simulink model "DFT_Stream_Ex1"  (R2022a)
settings: Solver=VariableStepAuto  StartTime=0.0  StopTime=0.6  RelTol=1e-3
undefined symbols (not defined in the file): None, S, vsva2197, xcvc1902
libraries: dspsrcs4 x1, aieDSP x1, vmcUtilities x1
settings Model: Creator=sdegala  LastModifiedBy=sdegala

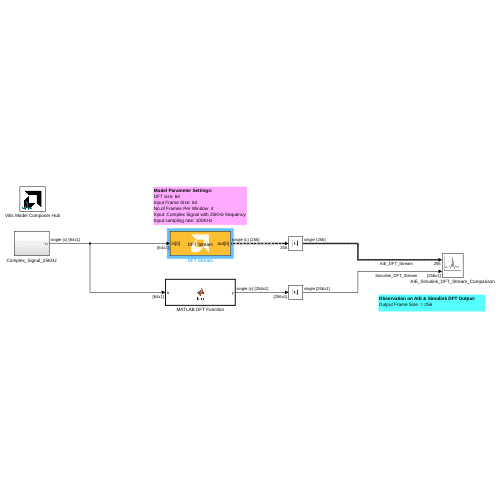
[thumbnail: Simulink's stored preview of the top-level diagram]
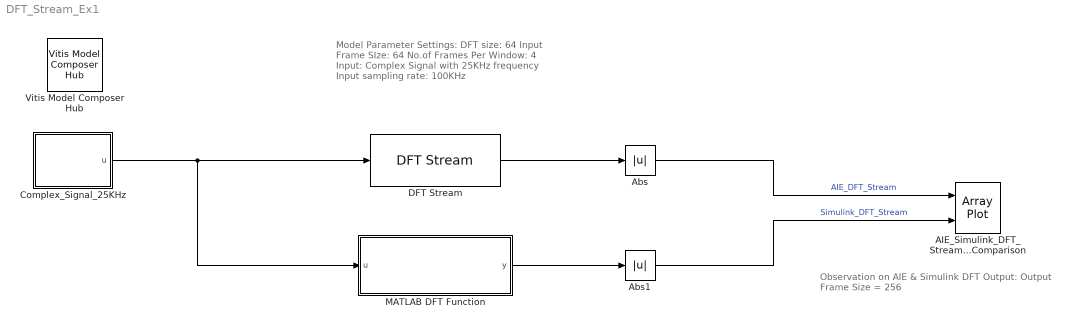
== system DFT_Stream_Ex1 ==
  note: Model Parameter Settings:
      | DFT size: 64
      | Input Frame SIze: 64
      | No.of Frames Per Window: 4
      | Input: Complex Signal with 25KHz frequency
      | Input sampling rate: 100KHz
  note: Observation on AIE & Simulink DFT Output:
      | Output Frame Size = 256
  AIE_Simulink_DFT_Stream_Comparison : ArrayPlot  NumInputPorts=2  WindowPosition=[5.000000,41.000000,1272.000000,651.000000,]  ScopeFrameLocation=window  YLimits=[-80,720]  ShowLegend=on
  Abs : Abs  SaturateOnIntegerOverflow=off
  Abs1 : Abs  SaturateOnIntegerOverflow=off
  Complex_Signal_25KHz : Subsystem
  DFT Stream : aieDSP/DFT Stream  data_type=cfloat  twiddle_type=cfloat  point_size=64  num_frames=4  shift_val=0  rnd_mode=Round symmetrical to infinity  sat_mode=0-None  casc_length=1  blockJsonConstraints=[]  blockJsonConstraintsInternal=[]  spec=vmc_stream_dft.json  SerializedMaskParamNames=[]  SerializedMaskParamValues=[]  SerializedMaskParamVisibilities=[]  block_type=DFT Stream  SerializedMaskParamDataypes=typename|typename|uint|uint|uint|uint|uint|uint  SerializedMaskParamEnumStrArr=0|0|0|0|0|Floor,Ceiling,Round to positive infinity,Round to negative infinity,Round symmetrical to infinity,Round symmetrical to zero,Round convergent to even,Round convergent to odd|0-None,1-Asymmetric,3-Symmetric|0  SerializedMaskParamEnumValArr=0|0|0|0|0|0,1,2,3,4,5,6,7|0,1,3|0  SerializedMaskParamVectorArr=0|0|0|0|0|0|0|0
  MATLAB DFT Function : MATLAB Function  TreatAsAtomicUnit=on
  Vitis Model Composer Hub : vmcUtilities/Vitis Model Composer Hub  Tag=genX  CodeGeneration=off  TargetDirectory=./code  ExportType=AI Engines  IpVendor=xilinx.com  IpLibrary=hls  IpVersion=1.0  IpHWLanguage=Verilog  AieCompilerOptions={}  AieSimulatorOptions={}  CreateTestbench=off  TestbenchStackSize=10  RunRtlSim=off  RunCSim=off  RunAieSim=off  AieSimTimeout=50000  RunAieSimProfiling=off  LaunchVitisAnalyzer=off  PlotOutput=off  RunX86Sim=off  X86SimTimeout=10  GenHwImage=off  GenLibadfXo=off  PlatformType=Not Specified  HwSystemType=Baremetal  HwValidationTarget=hw  ProjDevice=xcvc1902-vsva2197-1LP-e-S  ProjDevicePart=xcvc1902-vsva2197-1LP-e-S  AIEType=AIE  SamplePeriod=-1  ClockFrequency=200  DataPathParallelism=1  xilinxfamily=versalaicore  part=xcvc1902  speed=-1LP-e-S  package=vsva2197  directory=./code  testbench=off  incr_netlist=off  synthesis_tool=Vivado  clock_wrapper=Clock Enables  dbl_ovrd=According to Block Masks  dcm_input_clock_period=10  sysclk_period=10  simulink_period=1  eval_field=0  LogFileName=''  NThreads=4
  wires:
  Complex_Signal_25KHz/1(u) -> DFT Stream/1, MATLAB DFT Function/1(u)
  DFT Stream/1 -> Abs/1
  Abs/1 -> AIE_Simulink_DFT_Stream_Comparison/1  "AIE_DFT_Stream"
  MATLAB DFT Function/1(y) -> Abs1/1
  Abs1/1 -> AIE_Simulink_DFT_Stream_Comparison/2  "Simulink_DFT_Stream"

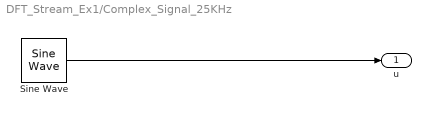
== system DFT_Stream_Ex1/Complex_Signal_25KHz ==
  Sine Wave : dspsrcs4/Sine Wave  Amplitude=10  Frequency=25e3  Phase=0  SampleMode=Discrete  OutComplex=Complex  CompMethod=Table lookup  TableSize=Speed  SampleTime=1/100e3  SamplesPerFrame=64  ResetState=Restart at time zero  OutputFrames=off  dataType=single  wordLen=16  udDataType=sfix(16)  fracBitsMode=User-defined  numFracBits=10  OutDataTypeStr=single  LastOutDataTypeStr=single
  u : Outport
  wires:
  Sine Wave/1 -> u/1

== matlab function DFT_Stream_Ex1/MATLAB DFT Function ==
  data: u input; y output

function y = fcn(u)

DFT_Size = 64; % DFT Size
FramesPerWindow = 4; %No.of Frames Per Window


X = single(complex(zeros(DFT_Size,FramesPerWindow)));

for m = 1:1:FramesPerWindow
for k = 0:DFT_Size-1
    for n = 0:DFT_Size-1
        X(k+1,m) = X(k+1,m) + u(n+1)*exp(-1i*2*pi*n*k/DFT_Size);
    end
end
end

y = reshape(X,DFT_Size*FramesPerWindow,1);
